simulink subsystem "Motoress"  (R2023b)
settings: Solver=VariableStepAuto  StartTime=0.0  StopTime=10.0  RelTol=1e-3
libraries: arduinolib x6, simulink x2
settings Model: Creator=marqu  LastModifiedBy=marqu

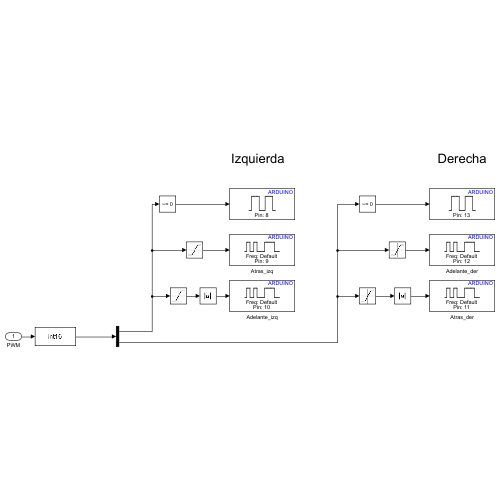
[thumbnail: Simulink's stored preview of the top-level diagram]
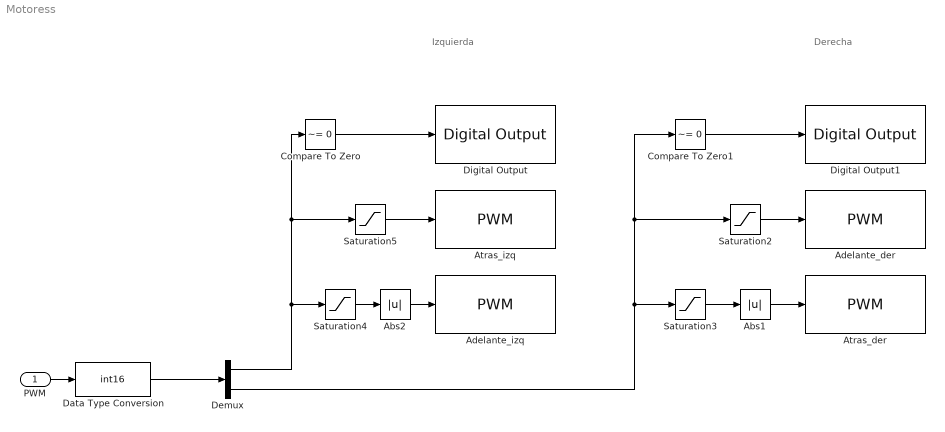
== system Motoress ==
  note: Derecha
  note: Izquierda
  PWM : Inport
  Abs1 : Abs  SaturateOnIntegerOverflow=off
  Abs2 : Abs  SaturateOnIntegerOverflow=off
  Adelante_der : arduinolib/PWM  pinNumber=12  frequencyType=Default  desiredFrequency=490.2  achievableFrequency=490.2
  Adelante_izq : arduinolib/PWM  pinNumber=9  frequencyType=Default  desiredFrequency=490.2  achievableFrequency=490.2
  Atras_der : arduinolib/PWM  pinNumber=11  frequencyType=Default  desiredFrequency=490.2  achievableFrequency=490.2
  Atras_izq : arduinolib/PWM  pinNumber=10  frequencyType=Default  desiredFrequency=490.2  achievableFrequency=490.2
  Compare To Zero : simulink/Logic and Bit Operations/Compare To Zero  relop=~=  OutDataTypeStr=boolean
  Compare To Zero1 : simulink/Logic and Bit Operations/Compare To Zero  relop=~=  OutDataTypeStr=boolean
  Data Type Conversion : DataTypeConversion  OutDataTypeStr=int16  SaturateOnIntegerOverflow=off  RndMeth=Floor
  Demux : Demux  Outputs=2
  Digital Output : arduinolib/Digital Output  pinNumber=8  Direction=output  blockPlatform=arduino
  Digital Output1 : arduinolib/Digital Output  pinNumber=13  Direction=output  blockPlatform=arduino
  Saturation2 : Saturate  UpperLimit=255  LowerLimit=0
  Saturation3 : Saturate  UpperLimit=0  LowerLimit=-255
  Saturation4 : Saturate  UpperLimit=0  LowerLimit=-255
  Saturation5 : Saturate  UpperLimit=255  LowerLimit=0
  wires:
  Data Type Conversion/1 -> Demux/1
  PWM/1 -> Data Type Conversion/1
  Compare To Zero1/1 -> Digital Output1/1
  Saturation2/1 -> Adelante_der/1
  Abs1/1 -> Atras_der/1
  Compare To Zero/1 -> Digital Output/1
  Saturation3/1 -> Abs1/1
  Saturation4/1 -> Abs2/1
  Abs2/1 -> Adelante_izq/1
  Saturation5/1 -> Atras_izq/1
  Demux/2 -> Compare To Zero1/1, Saturation2/1, Saturation3/1
  Demux/1 -> Saturation4/1, Saturation5/1, Compare To Zero/1
